simulink model "TBCC_Dyn"  (Simulink 10.0)
settings: Solver=VariableStepAuto  StartTime=0.0  StopTime=MWS.in.SimTime  FixedStep=MWS.Solve.T  RelTol=1e-3
values from neighbouring files (symbols this model uses):
  MWS = setup_Inlet(MWS)    [TBCC_setup_everything.m]
undefined symbols (not defined in the file or in its folder): combustion, diffuser, g, gama_ho, inlet_v, L_ho, nozzle, Pa, Pc_ho, R, R_ho, r_ho, stripchar_TMATS, Tc_ho, Wt_ho
libraries: Lib_Solve_ModelSource_TMATS x10, simulink_extras x7, Lib_Cntrl_FirstOrderSensor_TMATS x2, Lib_Solve_OuterLoopIntegrator_TMATS x2, Lib_Cntrl_SimplePIcontroller_TMATS x2, Lib_Turbo_Ambient_TMATS x2, Lib_Turbo_Burner_TMATS x2, Lib_Turbo_Compressor_TMATS x2, Lib_Turbo_Duct_TMATS x2, Lib_Turbo_Inlet_TMATS x2, Lib_Turbo_Nozzle_TMATS x2, Lib_Turbo_Shaft_TMATS x2
(part 2 of 2)

== system TBCC_Dyn/涡喷发动机结构模型/Iterative NR Solver w JacobianCalc/NRwCond ==
  note: Enable NR when conditions are not met
      | and Jacobian Calculator is not active
  f(x) : Inport  PortDimensions=length(SNR_IC_M)
  JC_Active : Inport  Port=2  PortDimensions=1
  inv(f'(x)) : Inport  Port=3  PortDimensions=[length(SNR_IC_M),length(SNR_IC_M)]
  Enable : EnablePort
  Iteration Conditions : Subsystem
  Logical Operator : Logic  Operator=NOT  AllPortsSameDT=off  OutDataTypeStr=boolean
  Logical Operator1 : Logic  AllPortsSameDT=off  OutDataTypeStr=boolean
  Newton Raphson Solver : Lib_NM_NewtonRaphsonSolver_TMATS/Newton Raphson Solver  NR_IC_M=ones(size(SNR_IC_M))  NR_dx_Lim_M=SNR_DX_M  NR_Mx_Lim_M=SNR_Mx_M./SNR_IC_M  NR_Mn_Lim_M=SNR_Mn_M./SNR_IC_M  BlkNm_M=double(gcb)
  Terminator : Terminator
  CCnd : Outport  PortDimensions=1
  x(n+1) : Outport  Port=2  PortDimensions=length(SNR_IC_M)
  wires:
  Iteration Conditions/1(Condition) -> CCnd/1, Logical Operator1/2
  Logical Operator/1 -> Logical Operator1/1
  Logical Operator1/1 -> Newton Raphson Solver/1
  inv(f'(x))/1 -> Newton Raphson Solver/2
  Newton Raphson Solver/1 -> Terminator/1
  Newton Raphson Solver/2 -> x(n+1)/1
  JC_Active/1 -> Logical Operator/1
  f(x)/1 -> Newton Raphson Solver/3, Iteration Conditions/1(f(x))

== system TBCC_Dyn/控制器B/If Action Subsystem1/If Action Subsystem1/If Action Subsystem1 ==
  In1 : Inport
  Action Port : ActionPort  ActionPortLabel=if(u1 <= 1)
  Transfer Fcn (with initial outputs) : simulink_extras/Additional Linear/Transfer Fcn (with initial outputs)  N=[1]  D="[10  1]"  Y0=3520  U0=0
  Out1 : Outport
  wires:
  In1/1 -> Transfer Fcn (with initial outputs)/1
  Transfer Fcn (with initial outputs)/1 -> Out1/1

== system TBCC_Dyn/控制器B/If Action Subsystem1/If Action Subsystem1/If Action Subsystem2 ==
  In1 : Inport
  Action Port : ActionPort  ActionPortLabel=else
  Transfer Fcn (with initial outputs) : simulink_extras/Additional Linear/Transfer Fcn (with initial outputs)  N=[1]  D="[10  1]"  Y0=7020  U0=0
  Out1 : Outport
  wires:
  Transfer Fcn (with initial outputs)/1 -> Out1/1
  In1/1 -> Transfer Fcn (with initial outputs)/1

== system TBCC_Dyn/涡喷发动机内部结构模型2/Iterative NR Solver w JacobianCalc/NRwCond/Iteration Conditions ==
  f(x) : Inport
  Abs : Abs
  Constant1 : Constant  Value=Cond_Limits_M
  Constant2 : Constant  Value=0
  Relational Operator : RelationalOperator  Operator=>  OutDataTypeStr=boolean  RndMeth=Nearest
  Relational Operator1 : RelationalOperator  Operator=>  OutDataTypeStr=boolean  RndMeth=Nearest
  Sum of Elements : Sum  Inputs=+
  Condition : Outport
  wires:
  Abs/1 -> Relational Operator/1
  Constant1/1 -> Relational Operator/2
  f(x)/1 -> Abs/1
  Relational Operator/1 -> Sum of Elements/1
  Constant2/1 -> Relational Operator1/2
  Sum of Elements/1 -> Relational Operator1/1
  Relational Operator1/1 -> Condition/1

== system TBCC_Dyn/涡喷发动机结构模型/Iterative NR Solver w JacobianCalc/NRwCond/Iteration Conditions ==
  f(x) : Inport
  Abs : Abs
  Constant1 : Constant  Value=Cond_Limits_M
  Constant2 : Constant  Value=0
  Relational Operator : RelationalOperator  Operator=>  OutDataTypeStr=boolean  RndMeth=Nearest
  Relational Operator1 : RelationalOperator  Operator=>  OutDataTypeStr=boolean  RndMeth=Nearest
  Sum of Elements : Sum  Inputs=+
  Condition : Outport
  wires:
  Abs/1 -> Relational Operator/1
  Constant1/1 -> Relational Operator/2
  f(x)/1 -> Abs/1
  Relational Operator/1 -> Sum of Elements/1
  Constant2/1 -> Relational Operator1/2
  Sum of Elements/1 -> Relational Operator1/1
  Relational Operator1/1 -> Condition/1
